simulink model "ymd"  (R2018b)
settings: configuration reference "Physics" (kept outside this file)
model workspace (MAT data in the model file):
  x0_initialstates = Simulink.Parameter
  x0_initialstates.Value = [0 0 0 0 0 0]
  x0_initialstates.DataType = 'auto'
  x0_initialstates.Dimensions = [1 6]
undefined symbols (not defined in the file): INIT__initialvalues__Vehicle_InitialVelocity_mps__1, tireRL__MFSIMPLE__r_tire_m, VEH__Aerodynamics__A_LongitudinalDrag_m2, VEH__Aerodynamics__cw_LongitudinalDrag, VEH__VehicleData__m_Vehicle_kg, VEH__VehicleData__w_TrackR_m, YMD_set_banking, YMD_set_bb, YMD_set_beta, YMD_set_delta, YMD_set_fx, YMD_set_tv, YMD_sim_model
libraries: simulink x3
settings Model: DataDictionary=vehicleparameters_vehdynsim.sldd  SimulationMode=accelerator  ParameterArgumentNames=x0_initialstates  OrderedModelArguments=off  Creator=wischnewski  LastModifiedBy=Freddy

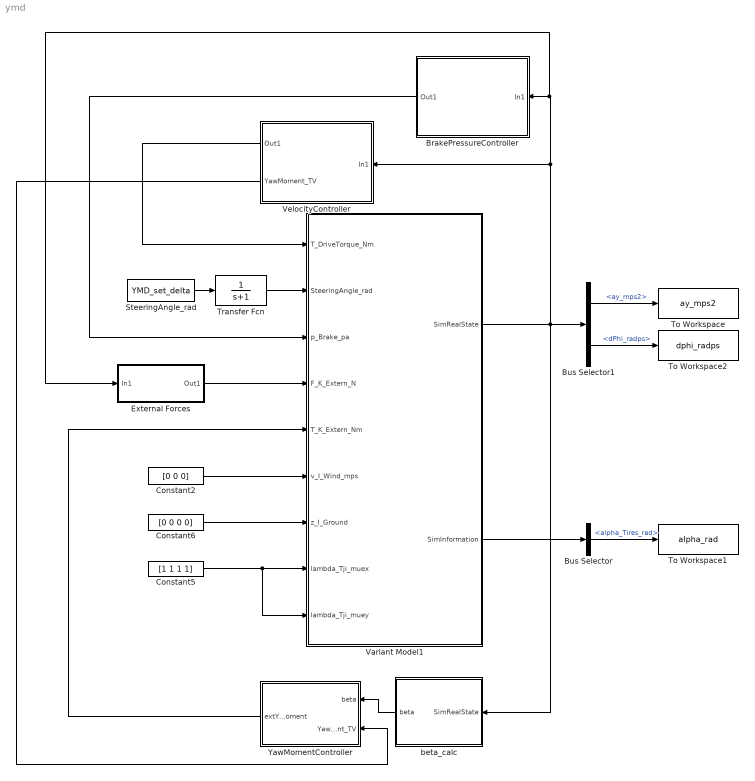
== system ymd ==
  BrakePressureController : Subsystem
  Bus Selector : BusSelector  OutputSignals=Wheel.alpha_Tires_rad
  Bus Selector1 : BusSelector  OutputSignals=ay_mps2,dPhi_radps
  Constant2 : Constant  Value=[0 0 0]
  Constant5 : Constant  Value=[1 1 1 1]
  Constant6 : Constant  Value=[0 0 0 0]
  External Forces : Subsystem
  SteeringAngle_rad : Constant  Value=YMD_set_delta
  To Workspace : ToWorkspace  VariableName=ay_mps2  SaveFormat=Timeseries  SampleTime=-1
  To Workspace1 : ToWorkspace  VariableName=alpha_rad  SaveFormat=Timeseries  SampleTime=-1
  To Workspace2 : ToWorkspace  VariableName=dphi_radps  SaveFormat=Timeseries  SampleTime=-1
  Transfer Fcn : TransferFcn  Denominator=[1 1]
  Variant Model1 : Subsystem  Variant=on
  VelocityController : Subsystem
  YawMomentController : Subsystem
  beta_calc : Subsystem
  wires:
  BrakePressureController/1(Out1) -> Variant Model1/3(p_Brake_pa)
  Variant Model1/1(SimRealState) -> beta_calc/1(SimRealState), Bus Selector1/1, External Forces/1(In1), BrakePressureController/1(In1), VelocityController/1(In1)
  Constant2/1 -> Variant Model1/6(v_I_Wind_mps)
  Constant6/1 -> Variant Model1/7(z_I_Ground)
  Constant5/1 -> Variant Model1/9(lambda_Tji_muey), Variant Model1/8(lambda_Tji_muex)
  beta_calc/1(beta) -> YawMomentController/1(beta)
  YawMomentController/1(extYawMoment) -> Variant Model1/5(T_K_Extern_Nm)
  VelocityController/1(Out1) -> Variant Model1/1(T_DriveTorque_Nm)
  External Forces/1(Out1) -> Variant Model1/4(F_K_Extern_N)
  VelocityController/2(YawMoment_TV) -> YawMomentController/2(YawMoment_TV)
  SteeringAngle_rad/1 -> Transfer Fcn/1
  Transfer Fcn/1 -> Variant Model1/2(SteeringAngle_rad)
  Variant Model1/2(SimInformation) -> Bus Selector/1
  Bus Selector/1 -> To Workspace1/1  "<alpha_Tires_rad>"
  Bus Selector1/1 -> To Workspace/1  "<ay_mps2>"
  Bus Selector1/2 -> To Workspace2/1  "<dPhi_radps>"

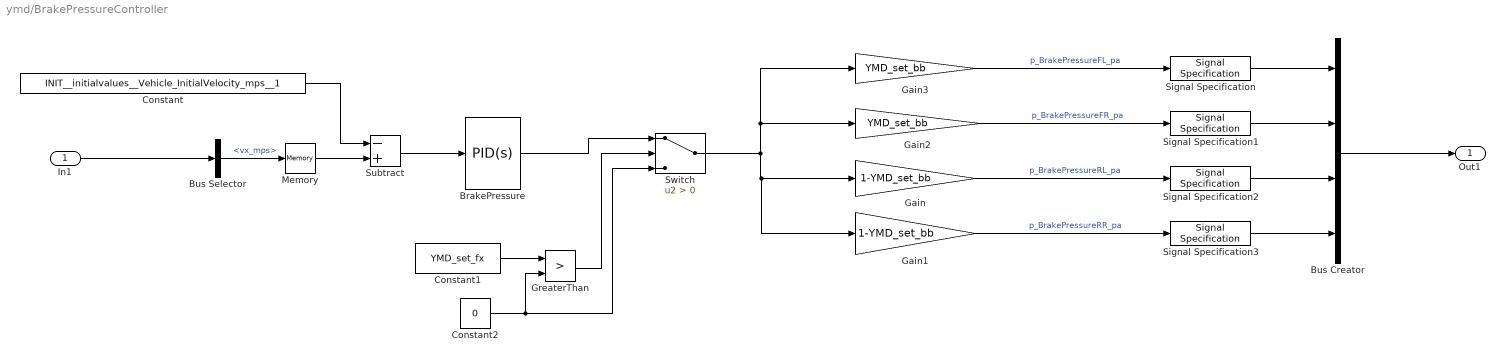
== system ymd/BrakePressureController ==
  In1 : Inport
  BrakePressure : simulink/Continuous/PID Controller  Controller=PID  Form=Parallel  TimeDomain=Continuous-time  SampleTime=-1  IntegratorMethod=Forward Euler  FilterMethod=Forward Euler  ControllerParametersSource=internal  P=4000000  I=50000000  D=0  UseFilter=on  N=100  TunerSelectOption=Transfer Function Based (PID Tuner App)  InitialConditionSource=internal  InitialConditionForIntegrator=0  InitialConditionForFilter=0  DifferentiatorICPrevScaledInput=0  ExternalReset=none  TrackingMode=off  Kt=1  LimitOutput=off  UpperSaturationLimit=inf  LowerSaturationLimit=-inf  LinearizeAsGain=on  AntiWindupMode=none  Kb=1  POutMin=[]  POutMax=[]  IOutMin=[]  IOutMax=[]  DOutMin=[]  DOutMax=[]  NOutMin=[]  NOutMax=[]  SumOutMin=[]  SumOutMax=[]  SaturationOutMin=[]  SaturationOutMax=[]  PParamMin=[]  PParamMax=[]  IParamMin=[]  IParamMax=[]  DParamMin=[]  DParamMax=[]  NParamMin=[]  NParamMax=[]  KbParamMin=[]  KbParamMax=[]  KtParamMin=[]  KtParamMax=[]  KbOutMin=[]  KbOutMax=[]  KtOutMin=[]  KtOutMax=[]  IntegratorOutMin=[]  IntegratorOutMax=[]  FilterOutMin=[]  FilterOutMax=[]  SumI1OutMin=[]  SumI1OutMax=[]  SumI2OutMin=[]  SumI2OutMax=[]  SumI3OutMin=[]  SumI3OutMax=[]  SumI4OutMin=[]  SumI4OutMax=[]  SumDOutMin=[]  SumDOutMax=[]  DifferentiatorOutMin=[]  DifferentiatorOutMax=[]  FilterDiffOutCoefMin=[]  FilterDiffOutCoefMax=[]  ReciprocalOutMin=[]  ReciprocalOutMax=[]  SumDenOutMin=[]  SumDenOutMax=[]  SumNumOutMin=[]  SumNumOutMax=[]  DivideOutMin=[]  DivideOutMax=[]  IntegratorContinuousStateAttributes=''  IntegratorStateMustResolveToSignalObject=off  IntegratorRTWStateStorageClass=Auto  FilterContinuousStateAttributes=''  FilterStateMustResolveToSignalObject=off  FilterRTWStateStorageClass=Auto  ParallelPVariant=InternalParameters  IdealPVariant=Disabled  IVariant=InternalParameters  DVariant=InternalParameters  IntegratorVariant=Continuous  SatVariant=Disabled  AWVariant=Passthrough  PCopyVariant=Disabled  TRVariant=Disabled  FdbkBlocksVariant=Forward  IdealPFdbkVariant=Disabled  SatFdbkVariant=Disabled  DerivativeFilterVariant=ContFilter  NVariant=InternalParameters  NCopyVariant=Disabled  FilterICVariant=InternalICsFilter  IntegratorICVariant=InternalICs  ExternalResetVariant=Disabled  TRSumVariant=Passthrough  SumFdbkVariant=Disabled  SumVariant=Sum_PID
  Bus Creator : BusCreator  Inputs=4
  Bus Selector : BusSelector  OutputSignals=vx_mps
  Constant : Constant  Value=INIT__initialvalues__Vehicle_InitialVelocity_mps__1
  Constant1 : Constant  Value=YMD_set_fx
  Constant2 : Constant  Value=0
  Gain : Gain  Gain=1-YMD_set_bb
  Gain1 : Gain  Gain=1-YMD_set_bb
  Gain2 : Gain  Gain=YMD_set_bb
  Gain3 : Gain  Gain=YMD_set_bb
  GreaterThan : RelationalOperator  Operator=>  OutDataTypeStr=boolean  RndMeth=Simplest
  Memory : Memory  InitialCondition=INIT__initialvalues__Vehicle_InitialVelocity_mps__1
  Signal Specification{,1..3} (4 alike) : SignalSpecification  Dimensions=1
  Subtract : Sum  Inputs=-+
  Switch : Switch  Criteria=u2 > Threshold
  Out1 : Outport
  wires:
  In1/1 -> Bus Selector/1
  Bus Selector/1 -> Memory/1  "<vx_mps>"
  Constant/1 -> Subtract/1
  Subtract/1 -> BrakePressure/1
  Bus Creator/1 -> Out1/1
  Gain1/1 -> Signal Specification3/1  "p_BrakePressureRR_pa"
  Gain/1 -> Signal Specification2/1  "p_BrakePressureRL_pa"
  Gain2/1 -> Signal Specification1/1  "p_BrakePressureFR_pa"
  Gain3/1 -> Signal Specification/1  "p_BrakePressureFL_pa"
  Signal Specification/1 -> Bus Creator/1
  Signal Specification1/1 -> Bus Creator/2
  Signal Specification2/1 -> Bus Creator/3
  Signal Specification3/1 -> Bus Creator/4
  BrakePressure/1 -> Switch/1
  Switch/1 -> Gain2/1, Gain3/1, Gain1/1, Gain/1
  GreaterThan/1 -> Switch/2
  Constant2/1 -> Switch/3, GreaterThan/2
  Constant1/1 -> GreaterThan/1
  Memory/1 -> Subtract/2

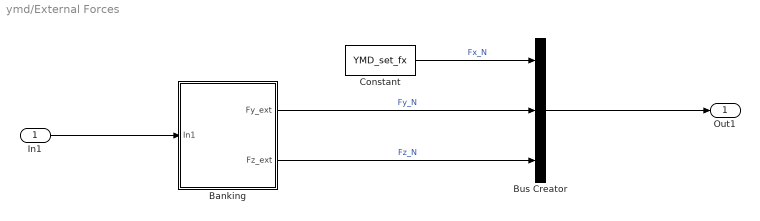
== system ymd/External Forces ==
  In1 : Inport
  Banking : Subsystem
  Bus Creator : BusCreator  Inputs=3
  Constant : Constant  Value=YMD_set_fx
  Out1 : Outport
  wires:
  Bus Creator/1 -> Out1/1
  Constant/1 -> Bus Creator/1  "Fx_N"
  In1/1 -> Banking/1(In1)
  Banking/1(Fy_ext) -> Bus Creator/2  "Fy_N"
  Banking/2(Fz_ext) -> Bus Creator/3  "Fz_N"

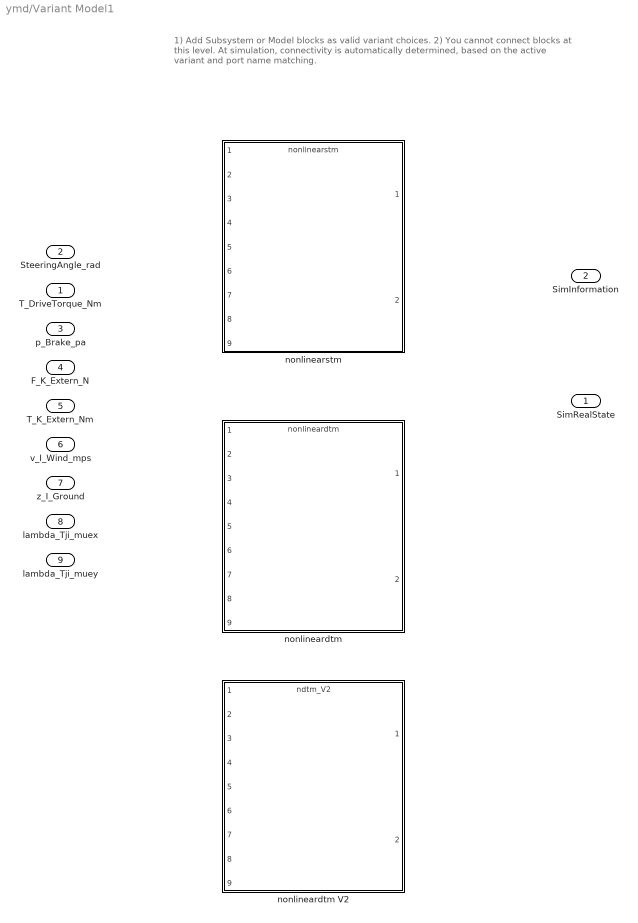
== system ymd/Variant Model1 ==
  note: 1) Add Subsystem or Model blocks as valid variant choices.
      | 2) You cannot connect blocks at this level. At simulation, connectivity is automatically
      | determined, based on the active variant and port name matching.
  T_DriveTorque_Nm : Inport
  SteeringAngle_rad : Inport  Port=2
  p_Brake_pa : Inport  Port=3
  F_K_Extern_N : Inport  Port=4  PortDimensions=3
  T_K_Extern_Nm : Inport  Port=5  PortDimensions=3
  v_I_Wind_mps : Inport  Port=6  PortDimensions=3
  z_I_Ground : Inport  Port=7  PortDimensions=4
  lambda_Tji_muex : Inport  Port=8  PortDimensions=4
  lambda_Tji_muey : Inport  Port=9  PortDimensions=4
  nonlineardtm : ModelReference  ModelNameDialog=nonlineardtm.slx  ParameterArgumentNames=x0_initialstates  ParameterArgumentValues=[0 0 0 0 0 -pi/2]  UsingDefaultArgumentValue=0  SimulationMode=Normal  VariantControl=YMD_sim_model==1  ModelReferenceVersion=1.737
  nonlineardtm V2 : ModelReference  ModelNameDialog=ndtm_V2.slx  ParameterArgumentNames=x0_initialstates  ParameterArgumentValues=[0 0 0 0 0 -pi/2]  UsingDefaultArgumentValue=0  SimulationMode=Normal  VariantControl=YMD_sim_model==3  ModelReferenceVersion=1.344
  nonlinearstm : ModelReference  ModelNameDialog=nonlinearstm.slx  ParameterArgumentNames=x0_positionstates  ParameterArgumentValues=[0 0 0]  UsingDefaultArgumentValue=0  SimulationMode=Normal  VariantControl=YMD_sim_model==2  ModelReferenceVersion=1.404
  SimRealState : Outport  OutDataTypeStr=Bus: SimRealState
  SimInformation : Outport  Port=2  OutDataTypeStr=Bus: SimInformation

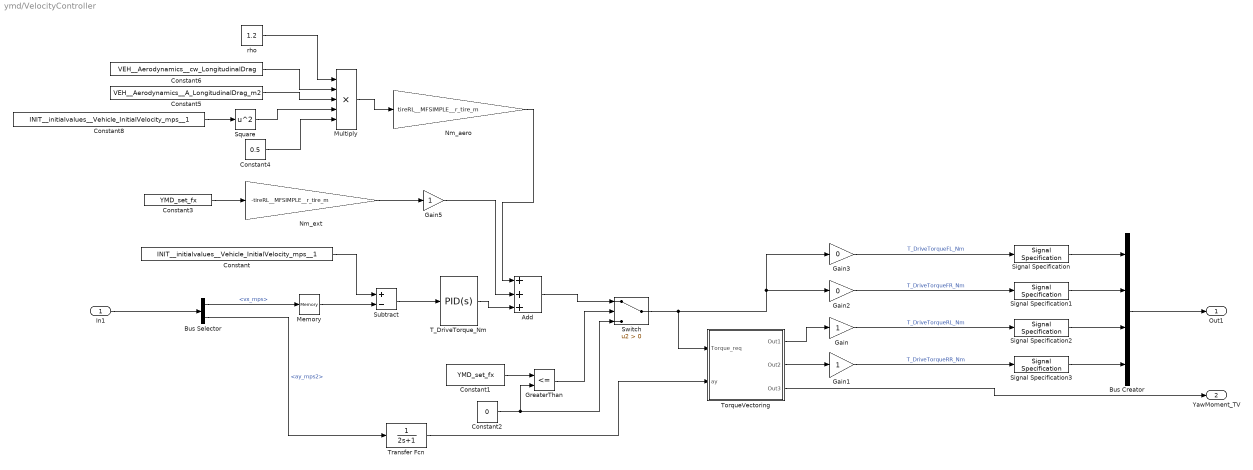
== system ymd/VelocityController ==
  In1 : Inport
  Add : Sum  Inputs=+++
  Bus Creator : BusCreator  Inputs=4
  Bus Selector : BusSelector  OutputSignals=vx_mps,ay_mps2
  Constant : Constant  Value=INIT__initialvalues__Vehicle_InitialVelocity_mps__1
  Constant1 : Constant  Value=YMD_set_fx
  Constant2 : Constant  Value=0
  Constant3 : Constant  Value=YMD_set_fx
  Constant4 : Constant  Value=0.5
  Constant5 : Constant  Value=VEH__Aerodynamics__A_LongitudinalDrag_m2
  Constant6 : Constant  Value=VEH__Aerodynamics__cw_LongitudinalDrag
  Constant8 : Constant  Value=INIT__initialvalues__Vehicle_InitialVelocity_mps__1
  Gain : Gain
  Gain1 : Gain
  Gain2 : Gain  Gain=0
  Gain3 : Gain  Gain=0
  Gain5 : Gain
  GreaterThan : RelationalOperator  Operator=<=  OutDataTypeStr=boolean  RndMeth=Simplest
  Memory : Memory  InitialCondition=INIT__initialvalues__Vehicle_InitialVelocity_mps__1
  Multiply : Product  Inputs=5
  Nm_aero : Gain  Gain=tireRL__MFSIMPLE__r_tire_m
  Nm_ext : Gain  Gain=-tireRL__MFSIMPLE__r_tire_m
  Signal Specification{,1..3} (4 alike) : SignalSpecification  Dimensions=1
  Square : Math  Operator=square  SaturateOnIntegerOverflow=on
  Subtract : Sum  Inputs=+-
  Switch : Switch  Criteria=u2 > Threshold
  T_DriveTorque_Nm : simulink/Continuous/PID Controller  Controller=PID  Form=Parallel  TimeDomain=Continuous-time  SampleTime=-1  IntegratorMethod=Forward Euler  FilterMethod=Forward Euler  ControllerParametersSource=internal  P=1000  I=1000  D=0  UseFilter=on  N=100  TunerSelectOption=Transfer Function Based (PID Tuner App)  InitialConditionSource=internal  InitialConditionForIntegrator=0  InitialConditionForFilter=0  DifferentiatorICPrevScaledInput=0  ExternalReset=none  TrackingMode=off  Kt=1  LimitOutput=on  UpperSaturationLimit=8000  LowerSaturationLimit=-8000  LinearizeAsGain=on  AntiWindupMode=none  Kb=1  POutMin=[]  POutMax=[]  IOutMin=[]  IOutMax=[]  DOutMin=[]  DOutMax=[]  NOutMin=[]  NOutMax=[]  SumOutMin=[]  SumOutMax=[]  SaturationOutMin=[]  SaturationOutMax=[]  PParamMin=[]  PParamMax=[]  IParamMin=[]  IParamMax=[]  DParamMin=[]  DParamMax=[]  NParamMin=[]  NParamMax=[]  KbParamMin=[]  KbParamMax=[]  KtParamMin=[]  KtParamMax=[]  KbOutMin=[]  KbOutMax=[]  KtOutMin=[]  KtOutMax=[]  IntegratorOutMin=[]  IntegratorOutMax=[]  FilterOutMin=[]  FilterOutMax=[]  SumI1OutMin=[]  SumI1OutMax=[]  SumI2OutMin=[]  SumI2OutMax=[]  SumI3OutMin=[]  SumI3OutMax=[]  SumI4OutMin=[]  SumI4OutMax=[]  SumDOutMin=[]  SumDOutMax=[]  DifferentiatorOutMin=[]  DifferentiatorOutMax=[]  FilterDiffOutCoefMin=[]  FilterDiffOutCoefMax=[]  ReciprocalOutMin=[]  ReciprocalOutMax=[]  SumDenOutMin=[]  SumDenOutMax=[]  SumNumOutMin=[]  SumNumOutMax=[]  DivideOutMin=[]  DivideOutMax=[]  IntegratorContinuousStateAttributes=''  IntegratorStateMustResolveToSignalObject=off  IntegratorRTWStateStorageClass=Auto  FilterContinuousStateAttributes=''  FilterStateMustResolveToSignalObject=off  FilterRTWStateStorageClass=Auto  ParallelPVariant=InternalParameters  IdealPVariant=Disabled  IVariant=InternalParameters  DVariant=InternalParameters  IntegratorVariant=Continuous  SatVariant=Enabled  AWVariant=Passthrough  PCopyVariant=Disabled  TRVariant=Disabled  FdbkBlocksVariant=Forward  IdealPFdbkVariant=Disabled  SatFdbkVariant=Disabled  DerivativeFilterVariant=ContFilter  NVariant=InternalParameters  NCopyVariant=Disabled  FilterICVariant=InternalICsFilter  IntegratorICVariant=InternalICs  ExternalResetVariant=Disabled  TRSumVariant=Passthrough  SumFdbkVariant=Disabled  SumVariant=Sum_PID
  TorqueVectoring : Subsystem
  Transfer Fcn : TransferFcn  Denominator=[2 1]
  rho : Constant  Value=1.2
  Out1 : Outport
  YawMoment_TV : Outport  Port=2
  wires:
  In1/1 -> Bus Selector/1
  Bus Selector/1 -> Memory/1  "<vx_mps>"
  Constant/1 -> Subtract/1
  Subtract/1 -> T_DriveTorque_Nm/1
  Bus Creator/1 -> Out1/1
  Gain1/1 -> Signal Specification3/1  "T_DriveTorqueRR_Nm"
  Gain/1 -> Signal Specification2/1  "T_DriveTorqueRL_Nm"
  Gain2/1 -> Signal Specification1/1  "T_DriveTorqueFR_Nm"
  Gain3/1 -> Signal Specification/1  "T_DriveTorqueFL_Nm"
  Signal Specification/1 -> Bus Creator/1
  Signal Specification1/1 -> Bus Creator/2
  Signal Specification2/1 -> Bus Creator/3
  Signal Specification3/1 -> Bus Creator/4
  Switch/1 -> TorqueVectoring/1(Torque_req), Gain2/1, Gain3/1
  Constant1/1 -> GreaterThan/1
  Constant2/1 -> Switch/3, GreaterThan/2
  GreaterThan/1 -> Switch/2
  Constant3/1 -> Nm_ext/1
  Add/1 -> Switch/1
  T_DriveTorque_Nm/1 -> Add/3
  Nm_ext/1 -> Gain5/1
  Constant8/1 -> Square/1
  Gain5/1 -> Add/2
  Multiply/1 -> Nm_aero/1
  Nm_aero/1 -> Add/1
  Constant4/1 -> Multiply/5
  Square/1 -> Multiply/4
  Constant5/1 -> Multiply/3
  Constant6/1 -> Multiply/2
  rho/1 -> Multiply/1
  Bus Selector/2 -> Transfer Fcn/1  "<ay_mps2>"
  TorqueVectoring/1(Out1) -> Gain/1
  TorqueVectoring/2(Out2) -> Gain1/1
  TorqueVectoring/3(Out3) -> YawMoment_TV/1
  Transfer Fcn/1 -> TorqueVectoring/2(ay)
  Memory/1 -> Subtract/2

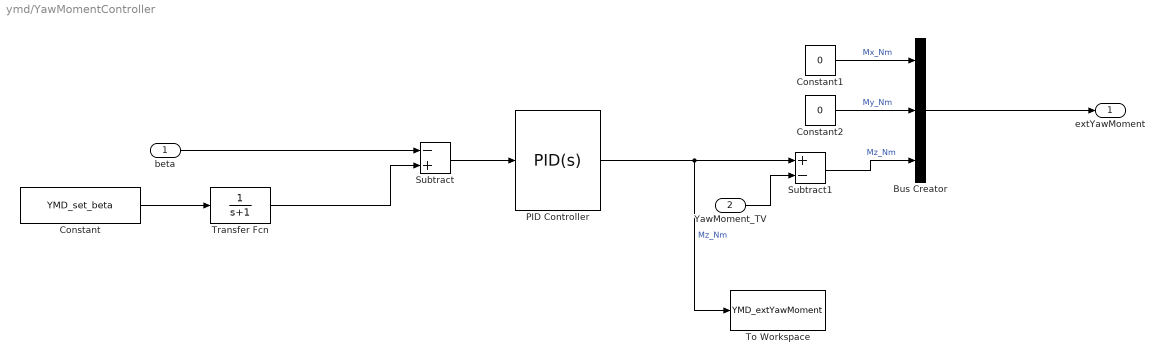
== system ymd/YawMomentController ==
  beta : Inport
  YawMoment_TV : Inport  Port=2
  Bus Creator : BusCreator  Inputs=3
  Constant : Constant  Value=YMD_set_beta
  Constant1 : Constant  Value=0
  Constant2 : Constant  Value=0
  PID Controller : simulink/Continuous/PID Controller  Controller=PID  Form=Parallel  TimeDomain=Continuous-time  SampleTime=-1  IntegratorMethod=Forward Euler  FilterMethod=Forward Euler  ControllerParametersSource=internal  P=400000  I=1000000  D=100000  UseFilter=on  N=15  TunerSelectOption=Transfer Function Based (PID Tuner App)  InitialConditionSource=internal  InitialConditionForIntegrator=0  InitialConditionForFilter=0  DifferentiatorICPrevScaledInput=0  ExternalReset=none  TrackingMode=off  Kt=1  LimitOutput=on  UpperSaturationLimit=50000  LowerSaturationLimit=-50000  LinearizeAsGain=on  AntiWindupMode=none  Kb=1  POutMin=[]  POutMax=[]  IOutMin=[]  IOutMax=[]  DOutMin=[]  DOutMax=[]  NOutMin=[]  NOutMax=[]  SumOutMin=[]  SumOutMax=[]  SaturationOutMin=[]  SaturationOutMax=[]  PParamMin=[]  PParamMax=[]  IParamMin=[]  IParamMax=[]  DParamMin=[]  DParamMax=[]  NParamMin=[]  NParamMax=[]  KbParamMin=[]  KbParamMax=[]  KtParamMin=[]  KtParamMax=[]  KbOutMin=[]  KbOutMax=[]  KtOutMin=[]  KtOutMax=[]  IntegratorOutMin=[]  IntegratorOutMax=[]  FilterOutMin=[]  FilterOutMax=[]  SumI1OutMin=[]  SumI1OutMax=[]  SumI2OutMin=[]  SumI2OutMax=[]  SumI3OutMin=[]  SumI3OutMax=[]  SumI4OutMin=[]  SumI4OutMax=[]  SumDOutMin=[]  SumDOutMax=[]  DifferentiatorOutMin=[]  DifferentiatorOutMax=[]  FilterDiffOutCoefMin=[]  FilterDiffOutCoefMax=[]  ReciprocalOutMin=[]  ReciprocalOutMax=[]  SumDenOutMin=[]  SumDenOutMax=[]  SumNumOutMin=[]  SumNumOutMax=[]  DivideOutMin=[]  DivideOutMax=[]  IntegratorContinuousStateAttributes=''  IntegratorStateMustResolveToSignalObject=off  IntegratorRTWStateStorageClass=Auto  FilterContinuousStateAttributes=''  FilterStateMustResolveToSignalObject=off  FilterRTWStateStorageClass=Auto  ParallelPVariant=InternalParameters  IdealPVariant=Disabled  IVariant=InternalParameters  DVariant=InternalParameters  IntegratorVariant=Continuous  SatVariant=Enabled  AWVariant=Passthrough  PCopyVariant=Disabled  TRVariant=Disabled  FdbkBlocksVariant=Forward  IdealPFdbkVariant=Disabled  SatFdbkVariant=Disabled  DerivativeFilterVariant=ContFilter  NVariant=InternalParameters  NCopyVariant=Disabled  FilterICVariant=InternalICsFilter  IntegratorICVariant=InternalICs  ExternalResetVariant=Disabled  TRSumVariant=Passthrough  SumFdbkVariant=Disabled  SumVariant=Sum_PID
  Subtract : Sum  Inputs=-+
  Subtract1 : Sum  Inputs=+-
  To Workspace : ToWorkspace  VariableName=YMD_extYawMoment  SaveFormat=Timeseries  SampleTime=-1
  Transfer Fcn : TransferFcn  Denominator=[1 1]
  extYawMoment : Outport
  wires:
  Constant/1 -> Transfer Fcn/1
  beta/1 -> Subtract/1
  Subtract/1 -> PID Controller/1
  PID Controller/1 -> Subtract1/1, To Workspace/1  "Mz_Nm"
  Bus Creator/1 -> extYawMoment/1
  Constant1/1 -> Bus Creator/1  "Mx_Nm"
  Constant2/1 -> Bus Creator/2  "My_Nm"
  Subtract1/1 -> Bus Creator/3  "Mz_Nm"
  YawMoment_TV/1 -> Subtract1/2
  Transfer Fcn/1 -> Subtract/2

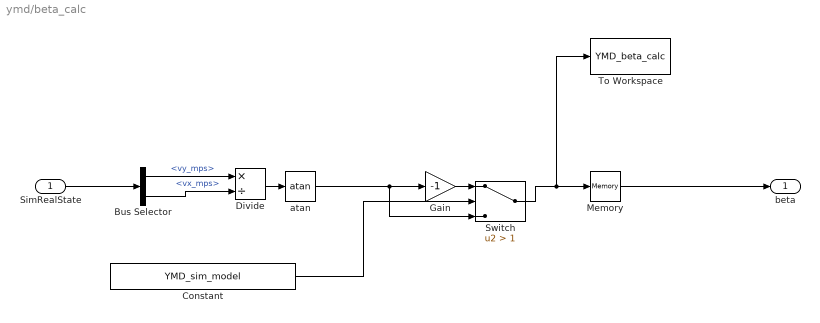
== system ymd/beta_calc ==
  SimRealState : Inport
  Bus Selector : BusSelector  OutputSignals=vy_mps,vx_mps
  Constant : Constant  Value=YMD_sim_model
  Divide : Product  Inputs=*/
  Gain : Gain  Gain=-1
  Memory : Memory
  Switch : Switch  Criteria=u2 > Threshold  Threshold=1
  To Workspace : ToWorkspace  VariableName=YMD_beta_calc  SaveFormat=Timeseries  SampleTime=-1
  atan : Trigonometry  Operator=atan
  beta : Outport
  wires:
  SimRealState/1 -> Bus Selector/1
  Bus Selector/1 -> Divide/1  "<vy_mps>"
  Bus Selector/2 -> Divide/2  "<vx_mps>"
  Divide/1 -> atan/1
  Memory/1 -> beta/1
  Constant/1 -> Switch/2
  Switch/1 -> To Workspace/1, Memory/1
  atan/1 -> Switch/3, Gain/1
  Gain/1 -> Switch/1

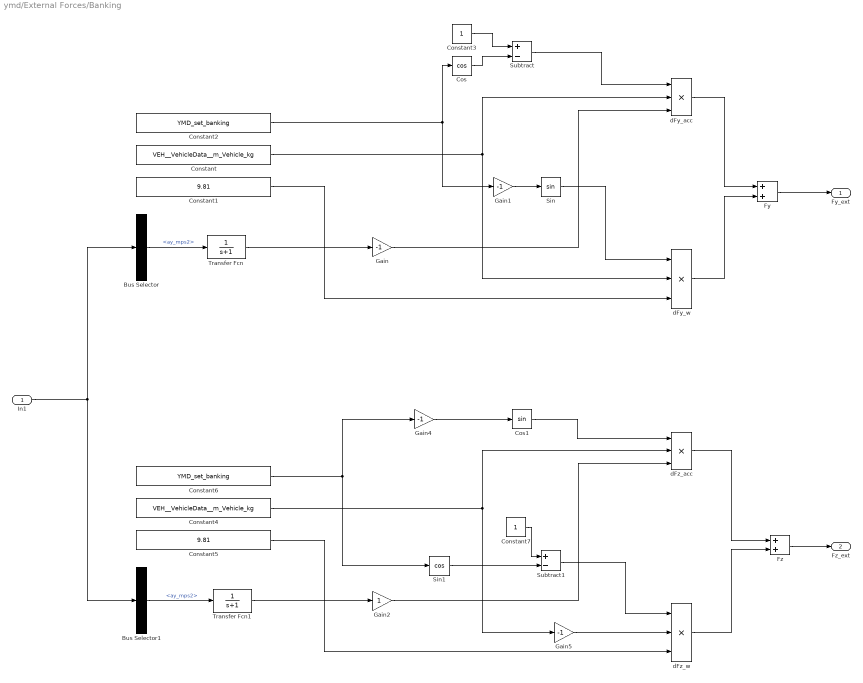
== system ymd/External Forces/Banking ==
  In1 : Inport
  Bus Selector : BusSelector  OutputSignals=ay_mps2
  Bus Selector1 : BusSelector  OutputSignals=ay_mps2
  Constant : Constant  Value=VEH__VehicleData__m_Vehicle_kg
  Constant1 : Constant  Value=9.81
  Constant2 : Constant  Value=YMD_set_banking
  Constant3 : Constant
  Constant4 : Constant  Value=VEH__VehicleData__m_Vehicle_kg
  Constant5 : Constant  Value=9.81
  Constant6 : Constant  Value=YMD_set_banking
  Constant7 : Constant
  Cos : Trigonometry  Operator=cos
  Cos1 : Trigonometry
  Fy : Sum
  Fz : Sum
  Gain{,1,4..5} (4 alike) : Gain  Gain=-1
  Gain2 : Gain
  Sin : Trigonometry
  Sin1 : Trigonometry  Operator=cos
  Subtract : Sum  Inputs=+-
  Subtract1 : Sum  Inputs=+-
  Transfer Fcn : TransferFcn  Denominator=[1 1]
  Transfer Fcn1 : TransferFcn  Denominator=[1 1]
  dFy_acc : Product  Inputs=3
  dFy_w : Product  Inputs=3
  dFz_acc : Product  Inputs=3
  dFz_w : Product  Inputs=3
  Fy_ext : Outport
  Fz_ext : Outport  Port=2
  wires:
  Bus Selector/1 -> Transfer Fcn/1  "<ay_mps2>"
  Gain/1 -> dFy_acc/3
  Constant/1 -> dFy_acc/2, dFy_w/2
  Constant3/1 -> Subtract/1
  Cos/1 -> Subtract/2
  Subtract/1 -> dFy_acc/1
  Constant1/1 -> dFy_w/3
  Gain1/1 -> Sin/1
  Sin/1 -> dFy_w/1
  In1/1 -> Bus Selector1/1, Bus Selector/1
  Constant5/1 -> dFz_w/3
  Constant4/1 -> dFz_acc/2, Gain5/1
  Gain2/1 -> dFz_acc/3
  Bus Selector1/1 -> Transfer Fcn1/1  "<ay_mps2>"
  Cos1/1 -> dFz_acc/1
  Gain4/1 -> Cos1/1
  Gain5/1 -> dFz_w/2
  Constant7/1 -> Subtract1/1
  Sin1/1 -> Subtract1/2
  Subtract1/1 -> dFz_w/1
  dFz_acc/1 -> Fz/1
  dFz_w/1 -> Fz/2
  dFy_acc/1 -> Fy/1
  dFy_w/1 -> Fy/2
  Fy/1 -> Fy_ext/1
  Fz/1 -> Fz_ext/1
  Constant2/1 -> Cos/1, Gain1/1
  Constant6/1 -> Gain4/1, Sin1/1
  Transfer Fcn/1 -> Gain/1
  Transfer Fcn1/1 -> Gain2/1

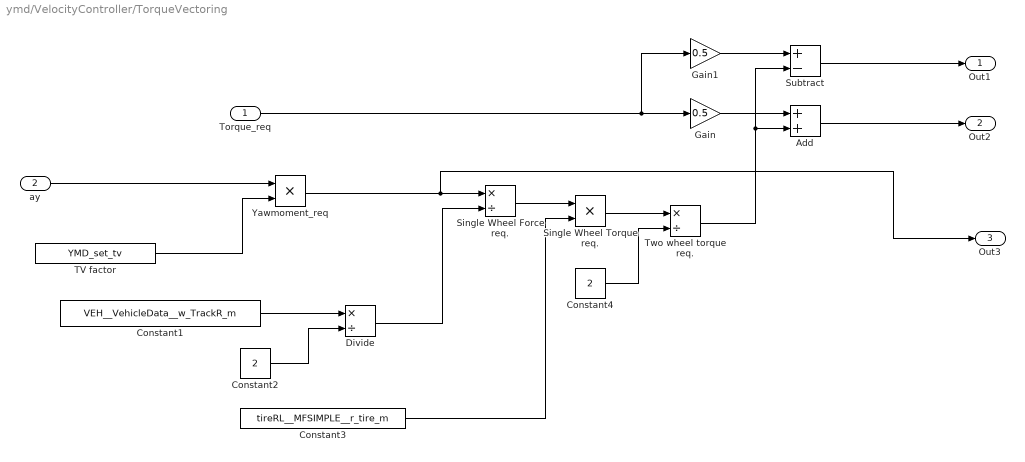
== system ymd/VelocityController/TorqueVectoring ==
  Torque_req : Inport
  ay : Inport  Port=2
  Add : Sum
  Constant1 : Constant  Value=VEH__VehicleData__w_TrackR_m
  Constant2 : Constant  Value=2
  Constant3 : Constant  Value=tireRL__MFSIMPLE__r_tire_m
  Constant4 : Constant  Value=2
  Divide : Product  Inputs=*/
  Gain : Gain  Gain=0.5
  Gain1 : Gain  Gain=0.5
  Single Wheel Force req. : Product  Inputs=*/
  Single Wheel Torque req. : Product
  Subtract : Sum  Inputs=+-
  TV factor : Constant  Value=YMD_set_tv
  Two wheel torque req. : Product  Inputs=*/
  Yawmoment_req : Product
  Out1 : Outport
  Out2 : Outport  Port=2
  Out3 : Outport  Port=3
  wires:
  TV factor/1 -> Yawmoment_req/2
  Constant1/1 -> Divide/1
  Constant2/1 -> Divide/2
  Divide/1 -> Single Wheel Force req./2
  Single Wheel Force req./1 -> Single Wheel Torque req./1
  Constant3/1 -> Single Wheel Torque req./2
  Single Wheel Torque req./1 -> Two wheel torque req./1
  Constant4/1 -> Two wheel torque req./2
  Torque_req/1 -> Gain1/1, Gain/1
  Gain/1 -> Add/1
  Two wheel torque req./1 -> Subtract/2, Add/2
  Gain1/1 -> Subtract/1
  Subtract/1 -> Out1/1
  Add/1 -> Out2/1
  Yawmoment_req/1 -> Out3/1, Single Wheel Force req./1
  ay/1 -> Yawmoment_req/1
